simulink model "doubleCond_strict"  (R2016b)
settings: Solver=VariableStepAuto  StartTime=0.0  StopTime=2  RelTol=1e-3
settings Model: Creator=live  LastModifiedBy=live

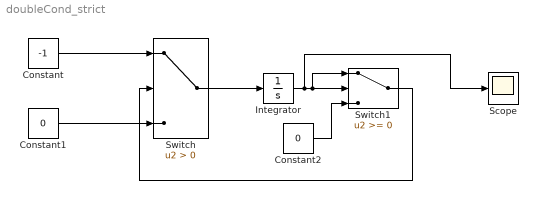
== system doubleCond_strict ==
  Constant : Constant  Value=-1
  Constant1 : Constant  Value=0
  Constant2 : Constant  Value=0
  Integrator : Integrator  InitialCondition=1
  Scope : Scope
  Switch : Switch  Criteria=u2 > Threshold
  Switch1 : Switch
  wires:
  Constant/1 -> Switch/1
  Constant1/1 -> Switch/3
  Switch/1 -> Integrator/1
  Integrator/1 -> Scope/1, Switch1/1, Switch1/2
  Constant2/1 -> Switch1/3
  Switch1/1 -> Switch/2
